simulink library "inp"  (R2021b)
settings: Solver=VariableStepAuto  StartTime=0.0  StopTime=10.0  RelTol=1e-3
undefined symbols (not defined in the file): C_TASK_5MS_S, FALSE, KINP_AcoreReadyToSlp_flg_ovrdflg, KINP_AcoreReadyToSlp_flg_ovrdval, KINP_AllowMovThd_OTA_enum_ovrdflg, KINP_AllowMovThd_OTA_enum_ovrdval, KINP_APSAngleTarget_Deg_ovrdflg, KINP_APSAngleTarget_Deg_ovrdval, KINP_APSDecReq_mps2_ovrdflg, KINP_APSDecReq_mps2_ovrdval, KINP_APSDecReqA_flg_ovrdflg, KINP_APSDecReqA_flg_ovrdval, KINP_APSDFLL_cm_ovrdflg, KINP_APSDFLL_cm_ovrdval, KINP_APSDFLR_cm_ovrdflg, KINP_APSDFLR_cm_ovrdval, KINP_APSDRLL_cm_ovrdflg, KINP_APSDRLL_cm_ovrdval, KINP_APSDRLR_cm_ovrdflg, KINP_APSDRLR_cm_ovrdval, KINP_APSExitCondition_enum_ovrdflg, KINP_APSExitCondition_enum_ovrdval, KINP_APSHWVer_enum_ovrdflg, KINP_APSHWVer_enum_ovrdval, KINP_APSProgressPCT_pct_ovrdflg, KINP_APSProgressPCT_pct_ovrdval, KINP_APSPwrReq_enum_ovrdflg, KINP_APSPwrReq_enum_ovrdval, KINP_APSReq_enum_ovrdflg, KINP_APSReq_enum_ovrdval, KINP_APSRQDisplay_enum_ovrdflg, KINP_APSRQDisplay_enum_ovrdval, KINP_APSRqEPASCtrl_flg_ovrdflg, KINP_APSRqEPASCtrl_flg_ovrdval, KINP_APSShiftPosnReq_enum_ovrdval, KINP_APSShiftPosnReq_enum_ovrflg, KINP_APSSpeedCMD_kph_ovrdval, KINP_APSSpeedCMD_kph_ovrflg, KINP_APSStaSystem_enum_ovrdflg, KINP_APSStaSystem_enum_ovrdval, KINP_APSSWVer_enum_ovrdflg, KINP_APSSWVer_enum_ovrdval, KINP_APSVMCReqA_flg_ovrdval, KINP_APSVMCReqA_flg_ovrflg, KINP_APSVRqEPASCtrl_flg_ovrdflg, KINP_APSVRqEPASCtrl_flg_ovrdval, KINP_AuxBattVolmV_mV_ovrdflg, KINP_AuxBattVolmV_mV_ovrdval, KINP_CAASSta_enum_ovrdflg, KINP_CAASSta_enum_ovrdval, KINP_CAASVMCReqA_flg_ovrdval, KINP_CAASVMCReqA_flg_ovrflg, KINP_CAN1BusOff_flg_ovrdflg, KINP_CAN1BusOff_flg_ovrdval, KINP_CAN2BusOff_flg_ovrdflg, KINP_CAN2BusOff_flg_ovrdval, KINP_CAN3BusOff_flg_ovrdflg, KINP_CAN3BusOff_flg_ovrdval, KINP_CAN4BusOff_flg_ovrdflg, KINP_CAN4BusOff_flg_ovrdval ... (+152)
libraries: FVT_lib x1035, hcu_lib x1
(part 25 of 33)

== system inp/INP/CAN4/SignalCheck/DKC1 ==
  BHAL_outputs : Inport
  inp_CanValid_bus : Inport  Port=2
  DKCKeyNumSta : FVT_lib/inp/can_signal_template  SystemSampleTime=-1  VariantActivationTime=update diagram  Latency=0  AutoFrameSizeCalculation=off
      link override defval: Value=KINP_DKCKeyNumSta_enum_defval
      link override ovrdflg: Value=KINP_DKCKeyNumSta_enum_ovrdflg
      link override ovrdval: Value=KINP_DKCKeyNumSta_enum_ovrdval
  DKCKeyTypeSta : FVT_lib/inp/can_signal_template  SystemSampleTime=-1  VariantActivationTime=update diagram  Latency=0  AutoFrameSizeCalculation=off
      link override defval: Value=KINP_DKCKeyTypeSta_enum_defval
      link override ovrdflg: Value=KINP_DKCKeyTypeSta_enum_ovrdflg
      link override ovrdval: Value=KINP_DKCKeyTypeSta_enum_ovrdval
  DKCPDkeyAreaRAPSSta : FVT_lib/inp/can_signal_template  SystemSampleTime=-1  VariantActivationTime=update diagram  Latency=0  AutoFrameSizeCalculation=off
      link override defval: Value=KINP_DKCPDkeyAreaRAPSSta_enum_defval
      link override ovrdflg: Value=KINP_DKCPDkeyAreaRAPSSta_enum_ovrdflg
      link override ovrdval: Value=KINP_DKCPDkeyAreaRAPSSta_enum_ovrdval
  DKCParkingModeCmd : FVT_lib/inp/can_signal_template  SystemSampleTime=-1  VariantActivationTime=update diagram  Latency=0  AutoFrameSizeCalculation=off
      link override defval: Value=KINP_DKCParkingModeCmd_enum_defval
      link override ovrdflg: Value=KINP_DKCParkingModeCmd_enum_ovrdflg
      link override ovrdval: Value=KINP_DKCParkingModeCmd_enum_ovrdval
  DKCReVehData : FVT_lib/inp/can_signal_template  SystemSampleTime=-1  VariantActivationTime=update diagram  Latency=0  AutoFrameSizeCalculation=off
      link override defval: Value=KINP_DKCReVehData_enum_defval
      link override ovrdflg: Value=KINP_DKCReVehData_enum_ovrdflg
      link override ovrdval: Value=KINP_DKCReVehData_enum_ovrdval
  PCommandToBCM : FVT_lib/inp/can_signal_template  SystemSampleTime=-1  VariantActivationTime=update diagram  Latency=0  AutoFrameSizeCalculation=off
      link override defval: Value=KINP_PCommandToBCM_enum_defval
      link override ovrdflg: Value=KINP_PCommandToBCM_enum_ovrdflg
      link override ovrdval: Value=KINP_PCommandToBCM_enum_ovrdval
  PCommandToPTG : FVT_lib/inp/can_signal_template  SystemSampleTime=-1  VariantActivationTime=update diagram  Latency=0  AutoFrameSizeCalculation=off
      link override defval: Value=KINP_PCommandToPTG_enum_defval
      link override ovrdflg: Value=KINP_PCommandToPTG_enum_ovrdflg
      link override ovrdval: Value=KINP_PCommandToPTG_enum_ovrdval
  PDKeyAreaLockUnlock : FVT_lib/inp/can_signal_template  SystemSampleTime=-1  VariantActivationTime=update diagram  Latency=0  AutoFrameSizeCalculation=off
      link override defval: Value=KINP_PDKeyAreaLockUnlock_enum_defval
      link override ovrdflg: Value=KINP_PDKeyAreaLockUnlock_enum_ovrdflg
      link override ovrdval: Value=KINP_PDKeyAreaLockUnlock_enum_ovrdval
  PDKeyAreaPS : FVT_lib/inp/can_signal_template  SystemSampleTime=-1  VariantActivationTime=update diagram  Latency=0  AutoFrameSizeCalculation=off
      link override defval: Value=KINP_PDKeyAreaPS_enum_defval
      link override ovrdflg: Value=KINP_PDKeyAreaPS_enum_ovrdflg
      link override ovrdval: Value=KINP_PDKeyAreaPS_enum_ovrdval
  PDKeyAreaPTG : FVT_lib/inp/can_signal_template  SystemSampleTime=-1  VariantActivationTime=update diagram  Latency=0  AutoFrameSizeCalculation=off
      link override defval: Value=KINP_PDKeyAreaPTG_enum_defval
      link override ovrdflg: Value=KINP_PDKeyAreaPTG_enum_ovrdflg
      link override ovrdval: Value=KINP_PDKeyAreaPTG_enum_ovrdval
  PDKeyWelcome : FVT_lib/inp/can_signal_template  SystemSampleTime=-1  VariantActivationTime=update diagram  Latency=0  AutoFrameSizeCalculation=off
      link override defval: Value=KINP_PDKeyWelcome_enum_defval
      link override ovrdflg: Value=KINP_PDKeyWelcome_enum_ovrdflg
      link override ovrdval: Value=KINP_PDKeyWelcome_enum_ovrdval
  PDkeyShowIVI : FVT_lib/inp/can_signal_template  SystemSampleTime=-1  VariantActivationTime=update diagram  Latency=0  AutoFrameSizeCalculation=off
      link override defval: Value=KINP_PDkeyShowIVI_enum_defval
      link override ovrdflg: Value=KINP_PDkeyShowIVI_enum_ovrdflg
      link override ovrdval: Value=KINP_PDkeyShowIVI_enum_ovrdval
  PKeyMiss : FVT_lib/inp/can_signal_template  SystemSampleTime=-1  VariantActivationTime=update diagram  Latency=0  AutoFrameSizeCalculation=off
      link override defval: Value=KINP_PKeyMiss_flg_defval
      link override ovrdflg: Value=KINP_PKeyMiss_flg_ovrdflg
      link override ovrdval: Value=KINP_PKeyMiss_flg_ovrdval
  PKeyMode : FVT_lib/inp/can_signal_template  SystemSampleTime=-1  VariantActivationTime=update diagram  Latency=0  AutoFrameSizeCalculation=off
      link override defval: Value=KINP_PKeyMode_enum_defval
      link override ovrdflg: Value=KINP_PKeyMode_enum_ovrdflg
      link override ovrdval: Value=KINP_PKeyMode_enum_ovrdval
  PUIDLowPower : FVT_lib/inp/can_signal_template  SystemSampleTime=-1  VariantActivationTime=update diagram  Latency=0  AutoFrameSizeCalculation=off
      link override defval: Value=KINP_PUIDLowPower_flg_defval
      link override ovrdflg: Value=KINP_PUIDLowPower_flg_ovrdflg
      link override ovrdval: Value=KINP_PUIDLowPower_flg_ovrdval
  Terminator_{1..15} (15 alike) : Terminator
  True_VHAL_DKCKeyNumSta_enum : Constant  Value=TRUE  OutDataTypeStr=boolean
  True_VHAL_DKCKeyTypeSta_enum : Constant  Value=TRUE  OutDataTypeStr=boolean
  True_VHAL_DKCPDkeyAreaRAPSSta_enum : Constant  Value=TRUE  OutDataTypeStr=boolean
  True_VHAL_DKCParkingModeCmd_enum : Constant  Value=TRUE  OutDataTypeStr=boolean
  True_VHAL_DKCReVehData_enum : Constant  Value=TRUE  OutDataTypeStr=boolean
  True_VHAL_PCommandToBCM_enum : Constant  Value=TRUE  OutDataTypeStr=boolean
  True_VHAL_PCommandToPTG_enum : Constant  Value=TRUE  OutDataTypeStr=boolean
  True_VHAL_PDKeyAreaLockUnlock_enum : Constant  Value=TRUE  OutDataTypeStr=boolean
  True_VHAL_PDKeyAreaPS_enum : Constant  Value=TRUE  OutDataTypeStr=boolean
  True_VHAL_PDKeyAreaPTG_enum : Constant  Value=TRUE  OutDataTypeStr=boolean
  True_VHAL_PDKeyWelcome_enum : Constant  Value=TRUE  OutDataTypeStr=boolean
  True_VHAL_PDkeyShowIVI_enum : Constant  Value=TRUE  OutDataTypeStr=boolean
  True_VHAL_PKeyMiss_flg : Constant  Value=TRUE  OutDataTypeStr=boolean
  True_VHAL_PKeyMode_enum : Constant  Value=TRUE  OutDataTypeStr=boolean
  True_VHAL_PUIDLowPower_flg : Constant  Value=TRUE  OutDataTypeStr=boolean
  slr1_{1..15} (15 alike) : BusSelector  OutputSignals=VINP_CANMsgValidDKC1_flg
  slr_VHAL_DKCKeyNumSta_enum : BusSelector  OutputSignals=VHAL_DKCKeyNumSta_enum
  slr_VHAL_DKCKeyTypeSta_enum : BusSelector  OutputSignals=VHAL_DKCKeyTypeSta_enum
  slr_VHAL_DKCPDkeyAreaRAPSSta_enum : BusSelector  OutputSignals=VHAL_DKCPDkeyAreaRAPSSta_enum
  slr_VHAL_DKCParkingModeCmd_enum : BusSelector  OutputSignals=VHAL_DKCParkingModeCmd_enum
  slr_VHAL_DKCReVehData_enum : BusSelector  OutputSignals=VHAL_DKCReVehData_enum
  slr_VHAL_PCommandToBCM_enum : BusSelector  OutputSignals=VHAL_PCommandToBCM_enum
  slr_VHAL_PCommandToPTG_enum : BusSelector  OutputSignals=VHAL_PCommandToPTG_enum
  slr_VHAL_PDKeyAreaLockUnlock_enum : BusSelector  OutputSignals=VHAL_PDKeyAreaLockUnlock_enum
  slr_VHAL_PDKeyAreaPS_enum : BusSelector  OutputSignals=VHAL_PDKeyAreaPS_enum
  slr_VHAL_PDKeyAreaPTG_enum : BusSelector  OutputSignals=VHAL_PDKeyAreaPTG_enum
  slr_VHAL_PDKeyWelcome_enum : BusSelector  OutputSignals=VHAL_PDKeyWelcome_enum
  slr_VHAL_PDkeyShowIVI_enum : BusSelector  OutputSignals=VHAL_PDkeyShowIVI_enum
  slr_VHAL_PKeyMiss_flg : BusSelector  OutputSignals=VHAL_PKeyMiss_flg
  slr_VHAL_PKeyMode_enum : BusSelector  OutputSignals=VHAL_PKeyMode_enum
  slr_VHAL_PUIDLowPower_flg : BusSelector  OutputSignals=VHAL_PUIDLowPower_flg
  VINP_DKCKeyNumSta_enum : Outport
  VINP_DKCKeyTypeSta_enum : Outport  Port=2
  VINP_DKCPDkeyAreaRAPSSta_enum : Outport  Port=3
  VINP_DKCParkingModeCmd_enum : Outport  Port=4
  VINP_DKCReVehData_enum : Outport  Port=5
  VINP_PCommandToBCM_enum : Outport  Port=6
  VINP_PCommandToPTG_enum : Outport  Port=7
  VINP_PDKeyAreaLockUnlock_enum : Outport  Port=8
  VINP_PDKeyAreaPS_enum : Outport  Port=9
  VINP_PDKeyAreaPTG_enum : Outport  Port=10
  VINP_PDKeyWelcome_enum : Outport  Port=11
  VINP_PDkeyShowIVI_enum : Outport  Port=12
  VINP_PKeyMiss_flg : Outport  Port=13
  VINP_PKeyMode_enum : Outport  Port=14
  VINP_PUIDLowPower_flg : Outport  Port=15
  wires:
  BHAL_outputs/1 -> [BHAL_outputs]
  inp_CanValid_bus/1 -> [inp_CanValid_bus]
  [BHAL_outputs] -> slr_VHAL_DKCKeyNumSta_enum/1
  slr_VHAL_DKCKeyNumSta_enum/1 -> DKCKeyNumSta/1  "<VHAL_DKCKeyNumSta_enum>"
  True_VHAL_DKCKeyNumSta_enum/1 -> DKCKeyNumSta/2
  [inp_CanValid_bus] -> slr1_1/1
  slr1_1/1 -> DKCKeyNumSta/3  "<VINP_CANMsgValidDKC1_flg>"
  DKCKeyNumSta/1 -> VINP_DKCKeyNumSta_enum/1  "VINP_DKCKeyNumSta_enum"
  DKCKeyNumSta/2 -> Terminator_1/1
  [BHAL_outputs] -> slr_VHAL_DKCKeyTypeSta_enum/1
  slr_VHAL_DKCKeyTypeSta_enum/1 -> DKCKeyTypeSta/1  "<VHAL_DKCKeyTypeSta_enum>"
  True_VHAL_DKCKeyTypeSta_enum/1 -> DKCKeyTypeSta/2
  [inp_CanValid_bus] -> slr1_2/1
  slr1_2/1 -> DKCKeyTypeSta/3  "<VINP_CANMsgValidDKC1_flg>"
  DKCKeyTypeSta/1 -> VINP_DKCKeyTypeSta_enum/1  "VINP_DKCKeyTypeSta_enum"
  DKCKeyTypeSta/2 -> Terminator_2/1
  [BHAL_outputs] -> slr_VHAL_DKCPDkeyAreaRAPSSta_enum/1
  slr_VHAL_DKCPDkeyAreaRAPSSta_enum/1 -> DKCPDkeyAreaRAPSSta/1  "<VHAL_DKCPDkeyAreaRAPSSta_enum>"
  True_VHAL_DKCPDkeyAreaRAPSSta_enum/1 -> DKCPDkeyAreaRAPSSta/2
  [inp_CanValid_bus] -> slr1_3/1
  slr1_3/1 -> DKCPDkeyAreaRAPSSta/3  "<VINP_CANMsgValidDKC1_flg>"
  DKCPDkeyAreaRAPSSta/1 -> VINP_DKCPDkeyAreaRAPSSta_enum/1  "VINP_DKCPDkeyAreaRAPSSta_enum"
  DKCPDkeyAreaRAPSSta/2 -> Terminator_3/1
  [BHAL_outputs] -> slr_VHAL_DKCParkingModeCmd_enum/1
  slr_VHAL_DKCParkingModeCmd_enum/1 -> DKCParkingModeCmd/1  "<VHAL_DKCParkingModeCmd_enum>"
  True_VHAL_DKCParkingModeCmd_enum/1 -> DKCParkingModeCmd/2
  [inp_CanValid_bus] -> slr1_4/1
  slr1_4/1 -> DKCParkingModeCmd/3  "<VINP_CANMsgValidDKC1_flg>"
  DKCParkingModeCmd/1 -> VINP_DKCParkingModeCmd_enum/1  "VINP_DKCParkingModeCmd_enum"
  DKCParkingModeCmd/2 -> Terminator_4/1
  [BHAL_outputs] -> slr_VHAL_DKCReVehData_enum/1
  slr_VHAL_DKCReVehData_enum/1 -> DKCReVehData/1  "<VHAL_DKCReVehData_enum>"
  True_VHAL_DKCReVehData_enum/1 -> DKCReVehData/2
  [inp_CanValid_bus] -> slr1_5/1
  slr1_5/1 -> DKCReVehData/3  "<VINP_CANMsgValidDKC1_flg>"
  DKCReVehData/1 -> VINP_DKCReVehData_enum/1  "VINP_DKCReVehData_enum"
  DKCReVehData/2 -> Terminator_5/1
  [BHAL_outputs] -> slr_VHAL_PCommandToBCM_enum/1
  slr_VHAL_PCommandToBCM_enum/1 -> PCommandToBCM/1  "<VHAL_PCommandToBCM_enum>"
  True_VHAL_PCommandToBCM_enum/1 -> PCommandToBCM/2
  [inp_CanValid_bus] -> slr1_6/1
  slr1_6/1 -> PCommandToBCM/3  "<VINP_CANMsgValidDKC1_flg>"
  PCommandToBCM/1 -> VINP_PCommandToBCM_enum/1  "VINP_PCommandToBCM_enum"
  PCommandToBCM/2 -> Terminator_6/1
  [BHAL_outputs] -> slr_VHAL_PCommandToPTG_enum/1
  slr_VHAL_PCommandToPTG_enum/1 -> PCommandToPTG/1  "<VHAL_PCommandToPTG_enum>"
  True_VHAL_PCommandToPTG_enum/1 -> PCommandToPTG/2
  [inp_CanValid_bus] -> slr1_7/1
  slr1_7/1 -> PCommandToPTG/3  "<VINP_CANMsgValidDKC1_flg>"
  PCommandToPTG/1 -> VINP_PCommandToPTG_enum/1  "VINP_PCommandToPTG_enum"
  PCommandToPTG/2 -> Terminator_7/1
  [BHAL_outputs] -> slr_VHAL_PDKeyAreaLockUnlock_enum/1
  slr_VHAL_PDKeyAreaLockUnlock_enum/1 -> PDKeyAreaLockUnlock/1  "<VHAL_PDKeyAreaLockUnlock_enum>"
  True_VHAL_PDKeyAreaLockUnlock_enum/1 -> PDKeyAreaLockUnlock/2
  [inp_CanValid_bus] -> slr1_8/1
  slr1_8/1 -> PDKeyAreaLockUnlock/3  "<VINP_CANMsgValidDKC1_flg>"
  PDKeyAreaLockUnlock/1 -> VINP_PDKeyAreaLockUnlock_enum/1  "VINP_PDKeyAreaLockUnlock_enum"
  PDKeyAreaLockUnlock/2 -> Terminator_8/1
  [BHAL_outputs] -> slr_VHAL_PDKeyAreaPS_enum/1
  slr_VHAL_PDKeyAreaPS_enum/1 -> PDKeyAreaPS/1  "<VHAL_PDKeyAreaPS_enum>"
  True_VHAL_PDKeyAreaPS_enum/1 -> PDKeyAreaPS/2
  [inp_CanValid_bus] -> slr1_9/1
  slr1_9/1 -> PDKeyAreaPS/3  "<VINP_CANMsgValidDKC1_flg>"
  PDKeyAreaPS/1 -> VINP_PDKeyAreaPS_enum/1  "VINP_PDKeyAreaPS_enum"
  PDKeyAreaPS/2 -> Terminator_9/1
  [BHAL_outputs] -> slr_VHAL_PDKeyAreaPTG_enum/1
  slr_VHAL_PDKeyAreaPTG_enum/1 -> PDKeyAreaPTG/1  "<VHAL_PDKeyAreaPTG_enum>"
  True_VHAL_PDKeyAreaPTG_enum/1 -> PDKeyAreaPTG/2
  [inp_CanValid_bus] -> slr1_10/1
  slr1_10/1 -> PDKeyAreaPTG/3  "<VINP_CANMsgValidDKC1_flg>"
  PDKeyAreaPTG/1 -> VINP_PDKeyAreaPTG_enum/1  "VINP_PDKeyAreaPTG_enum"
  PDKeyAreaPTG/2 -> Terminator_10/1
  [BHAL_outputs] -> slr_VHAL_PDKeyWelcome_enum/1
  slr_VHAL_PDKeyWelcome_enum/1 -> PDKeyWelcome/1  "<VHAL_PDKeyWelcome_enum>"
  True_VHAL_PDKeyWelcome_enum/1 -> PDKeyWelcome/2
  [inp_CanValid_bus] -> slr1_11/1
  slr1_11/1 -> PDKeyWelcome/3  "<VINP_CANMsgValidDKC1_flg>"
  PDKeyWelcome/1 -> VINP_PDKeyWelcome_enum/1  "VINP_PDKeyWelcome_enum"
  PDKeyWelcome/2 -> Terminator_11/1
  [BHAL_outputs] -> slr_VHAL_PDkeyShowIVI_enum/1
  slr_VHAL_PDkeyShowIVI_enum/1 -> PDkeyShowIVI/1  "<VHAL_PDkeyShowIVI_enum>"
  True_VHAL_PDkeyShowIVI_enum/1 -> PDkeyShowIVI/2
  [inp_CanValid_bus] -> slr1_12/1
  slr1_12/1 -> PDkeyShowIVI/3  "<VINP_CANMsgValidDKC1_flg>"
  PDkeyShowIVI/1 -> VINP_PDkeyShowIVI_enum/1  "VINP_PDkeyShowIVI_enum"
  PDkeyShowIVI/2 -> Terminator_12/1
  [BHAL_outputs] -> slr_VHAL_PKeyMiss_flg/1
  slr_VHAL_PKeyMiss_flg/1 -> PKeyMiss/1  "<VHAL_PKeyMiss_flg>"
  True_VHAL_PKeyMiss_flg/1 -> PKeyMiss/2
  [inp_CanValid_bus] -> slr1_13/1
  slr1_13/1 -> PKeyMiss/3  "<VINP_CANMsgValidDKC1_flg>"
  PKeyMiss/1 -> VINP_PKeyMiss_flg/1  "VINP_PKeyMiss_flg"
  PKeyMiss/2 -> Terminator_13/1
  [BHAL_outputs] -> slr_VHAL_PKeyMode_enum/1
  slr_VHAL_PKeyMode_enum/1 -> PKeyMode/1  "<VHAL_PKeyMode_enum>"
  True_VHAL_PKeyMode_enum/1 -> PKeyMode/2
  [inp_CanValid_bus] -> slr1_14/1
  slr1_14/1 -> PKeyMode/3  "<VINP_CANMsgValidDKC1_flg>"
  PKeyMode/1 -> VINP_PKeyMode_enum/1  "VINP_PKeyMode_enum"
  PKeyMode/2 -> Terminator_14/1
  [BHAL_outputs] -> slr_VHAL_PUIDLowPower_flg/1
  slr_VHAL_PUIDLowPower_flg/1 -> PUIDLowPower/1  "<VHAL_PUIDLowPower_flg>"
  True_VHAL_PUIDLowPower_flg/1 -> PUIDLowPower/2
  [inp_CanValid_bus] -> slr1_15/1
  slr1_15/1 -> PUIDLowPower/3  "<VINP_CANMsgValidDKC1_flg>"
  PUIDLowPower/1 -> VINP_PUIDLowPower_flg/1  "VINP_PUIDLowPower_flg"
  PUIDLowPower/2 -> Terminator_15/1

== system inp/INP/CAN4/SignalCheck/DKC2 ==
  BHAL_outputs : Inport
  inp_CanValid_bus : Inport  Port=2
  EncryptionDATA063 : FVT_lib/inp/can_signal_template  SystemSampleTime=-1  VariantActivationTime=update diagram  Latency=0  AutoFrameSizeCalculation=off
      link override defval: Value=KINP_EncryptionDATA063_enum_defval
      link override ovrdflg: Value=KINP_EncryptionDATA063_enum_ovrdflg
      link override ovrdval: Value=KINP_EncryptionDATA063_enum_ovrdval
  EncryptionDATA64127 : FVT_lib/inp/can_signal_template  SystemSampleTime=-1  VariantActivationTime=update diagram  Latency=0  AutoFrameSizeCalculation=off
      link override defval: Value=KINP_EncryptionDATA64127_enum_defval
      link override ovrdflg: Value=KINP_EncryptionDATA64127_enum_ovrdflg
      link override ovrdval: Value=KINP_EncryptionDATA64127_enum_ovrdval
  RandomNumberX : FVT_lib/inp/can_signal_template  SystemSampleTime=-1  VariantActivationTime=update diagram  Latency=0  AutoFrameSizeCalculation=off
      link override defval: Value=KINP_RandomNumberX_enum_defval
      link override ovrdflg: Value=KINP_RandomNumberX_enum_ovrdflg
      link override ovrdval: Value=KINP_RandomNumberX_enum_ovrdval
  Terminator_1 : Terminator
  Terminator_2 : Terminator
  Terminator_3 : Terminator
  True_VHAL_EncryptionDATA063_enum : Constant  Value=TRUE  OutDataTypeStr=boolean
  True_VHAL_EncryptionDATA64127_enum : Constant  Value=TRUE  OutDataTypeStr=boolean
  True_VHAL_RandomNumberX_enum : Constant  Value=TRUE  OutDataTypeStr=boolean
  slr1_1 : BusSelector  OutputSignals=VINP_CANMsgValidDKC2_flg
  slr1_2 : BusSelector  OutputSignals=VINP_CANMsgValidDKC2_flg
  slr1_3 : BusSelector  OutputSignals=VINP_CANMsgValidDKC2_flg
  slr_VHAL_EncryptionDATA063_enum : BusSelector  OutputSignals=VHAL_EncryptionDATA063_enum
  slr_VHAL_EncryptionDATA64127_enum : BusSelector  OutputSignals=VHAL_EncryptionDATA64127_enum
  slr_VHAL_RandomNumberX_enum : BusSelector  OutputSignals=VHAL_RandomNumberX_enum
  VINP_EncryptionDATA063_enum : Outport
  VINP_EncryptionDATA64127_enum : Outport  Port=2
  VINP_RandomNumberX_enum : Outport  Port=3
  wires:
  BHAL_outputs/1 -> [BHAL_outputs]
  inp_CanValid_bus/1 -> [inp_CanValid_bus]
  [BHAL_outputs] -> slr_VHAL_EncryptionDATA063_enum/1
  slr_VHAL_EncryptionDATA063_enum/1 -> EncryptionDATA063/1  "<VHAL_EncryptionDATA063_enum>"
  True_VHAL_EncryptionDATA063_enum/1 -> EncryptionDATA063/2
  [inp_CanValid_bus] -> slr1_1/1
  slr1_1/1 -> EncryptionDATA063/3  "<VINP_CANMsgValidDKC2_flg>"
  EncryptionDATA063/1 -> VINP_EncryptionDATA063_enum/1  "VINP_EncryptionDATA063_enum"
  EncryptionDATA063/2 -> Terminator_1/1
  [BHAL_outputs] -> slr_VHAL_EncryptionDATA64127_enum/1
  slr_VHAL_EncryptionDATA64127_enum/1 -> EncryptionDATA64127/1  "<VHAL_EncryptionDATA64127_enum>"
  True_VHAL_EncryptionDATA64127_enum/1 -> EncryptionDATA64127/2
  [inp_CanValid_bus] -> slr1_2/1
  slr1_2/1 -> EncryptionDATA64127/3  "<VINP_CANMsgValidDKC2_flg>"
  EncryptionDATA64127/1 -> VINP_EncryptionDATA64127_enum/1  "VINP_EncryptionDATA64127_enum"
  EncryptionDATA64127/2 -> Terminator_2/1
  [BHAL_outputs] -> slr_VHAL_RandomNumberX_enum/1
  slr_VHAL_RandomNumberX_enum/1 -> RandomNumberX/1  "<VHAL_RandomNumberX_enum>"
  True_VHAL_RandomNumberX_enum/1 -> RandomNumberX/2
  [inp_CanValid_bus] -> slr1_3/1
  slr1_3/1 -> RandomNumberX/3  "<VINP_CANMsgValidDKC2_flg>"
  RandomNumberX/1 -> VINP_RandomNumberX_enum/1  "VINP_RandomNumberX_enum"
  RandomNumberX/2 -> Terminator_3/1

== system inp/INP/CAN4/SignalCheck/PTG1 ==
  BHAL_outputs : Inport
  inp_CanValid_bus : Inport  Port=2
  PTGActiveSta : FVT_lib/inp/can_signal_template  SystemSampleTime=-1  VariantActivationTime=update diagram  Latency=0  AutoFrameSizeCalculation=off
      link override defval: Value=KINP_PTGActiveSta_enum_defval
      link override ovrdflg: Value=KINP_PTGActiveSta_enum_ovrdflg
      link override ovrdval: Value=KINP_PTGActiveSta_enum_ovrdval
  PTGAutoStaus : FVT_lib/inp/can_signal_template  SystemSampleTime=-1  VariantActivationTime=update diagram  Latency=0  AutoFrameSizeCalculation=off
      link override defval: Value=KINP_PTGAutoStaus_flg_defval
      link override ovrdflg: Value=KINP_PTGAutoStaus_flg_ovrdflg
      link override ovrdval: Value=KINP_PTGAutoStaus_flg_ovrdval
  PTGExist : FVT_lib/inp/can_signal_template  SystemSampleTime=-1  VariantActivationTime=update diagram  Latency=0  AutoFrameSizeCalculation=off
      link override defval: Value=KINP_PTGExist_flg_defval
      link override ovrdflg: Value=KINP_PTGExist_flg_ovrdflg
      link override ovrdval: Value=KINP_PTGExist_flg_ovrdval
  PTGHWVer : FVT_lib/inp/can_signal_template  SystemSampleTime=-1  VariantActivationTime=update diagram  Latency=0  AutoFrameSizeCalculation=off
      link override defval: Value=KINP_PTGHWVer_enum_defval
      link override ovrdflg: Value=KINP_PTGHWVer_enum_ovrdflg
      link override ovrdval: Value=KINP_PTGHWVer_enum_ovrdval
  PTGInnerSW2 : FVT_lib/inp/can_signal_template  SystemSampleTime=-1  VariantActivationTime=update diagram  Latency=0  AutoFrameSizeCalculation=off
      link override defval: Value=KINP_PTGInnerSW2_enum_defval
      link override ovrdflg: Value=KINP_PTGInnerSW2_enum_ovrdflg
      link override ovrdval: Value=KINP_PTGInnerSW2_enum_ovrdval
  PTGIsSetHeight : FVT_lib/inp/can_signal_template  SystemSampleTime=-1  VariantActivationTime=update diagram  Latency=0  AutoFrameSizeCalculation=off
      link override defval: Value=KINP_PTGIsSetHeight_flg_defval
      link override ovrdflg: Value=KINP_PTGIsSetHeight_flg_ovrdflg
      link override ovrdval: Value=KINP_PTGIsSetHeight_flg_ovrdval
  PTGOpenRatio : FVT_lib/inp/can_signal_template  SystemSampleTime=-1  VariantActivationTime=update diagram  Latency=0  AutoFrameSizeCalculation=off
      link override defval: Value=KINP_PTGOpenRatio_pct_defval
      link override ovrdflg: Value=KINP_PTGOpenRatio_pct_ovrdflg
      link override ovrdval: Value=KINP_PTGOpenRatio_pct_ovrdval
  PTGRDILSta : FVT_lib/inp/can_signal_template  SystemSampleTime=-1  VariantActivationTime=update diagram  Latency=0  AutoFrameSizeCalculation=off
      link override defval: Value=KINP_PTGRDILSta_enum_defval
      link override ovrdflg: Value=KINP_PTGRDILSta_enum_ovrdflg
      link override ovrdval: Value=KINP_PTGRDILSta_enum_ovrdval
  PTGSWVer : FVT_lib/inp/can_signal_template  SystemSampleTime=-1  VariantActivationTime=update diagram  Latency=0  AutoFrameSizeCalculation=off
      link override defval: Value=KINP_PTGSWVer_enum_defval
      link override ovrdflg: Value=KINP_PTGSWVer_enum_ovrdflg
      link override ovrdval: Value=KINP_PTGSWVer_enum_ovrdval
  PTGSysSta : FVT_lib/inp/can_signal_template  SystemSampleTime=-1  VariantActivationTime=update diagram  Latency=0  AutoFrameSizeCalculation=off
      link override defval: Value=KINP_PTGSysSta_enum_defval
      link override ovrdflg: Value=KINP_PTGSysSta_enum_ovrdflg
      link override ovrdval: Value=KINP_PTGSysSta_enum_ovrdval
  Terminator_{1..10} (10 alike) : Terminator
  True_VHAL_PTGActiveSta_enum : Constant  Value=TRUE  OutDataTypeStr=boolean
  True_VHAL_PTGAutoStaus_flg : Constant  Value=TRUE  OutDataTypeStr=boolean
  True_VHAL_PTGExist_flg : Constant  Value=TRUE  OutDataTypeStr=boolean
  True_VHAL_PTGHWVer_enum : Constant  Value=TRUE  OutDataTypeStr=boolean
  True_VHAL_PTGInnerSW2_enum : Constant  Value=TRUE  OutDataTypeStr=boolean
  True_VHAL_PTGIsSetHeight_flg : Constant  Value=TRUE  OutDataTypeStr=boolean
  True_VHAL_PTGOpenRatio_pct : Constant  Value=TRUE  OutDataTypeStr=boolean
  True_VHAL_PTGRDILSta_enum : Constant  Value=TRUE  OutDataTypeStr=boolean
  True_VHAL_PTGSWVer_enum : Constant  Value=TRUE  OutDataTypeStr=boolean
  True_VHAL_PTGSysSta_enum : Constant  Value=TRUE  OutDataTypeStr=boolean
  slr1_{1..10} (10 alike) : BusSelector  OutputSignals=VINP_CANMsgValidPTG1_flg
  slr_VHAL_PTGActiveSta_enum : BusSelector  OutputSignals=VHAL_PTGActiveSta_enum
  slr_VHAL_PTGAutoStaus_flg : BusSelector  OutputSignals=VHAL_PTGAutoStaus_flg
  slr_VHAL_PTGExist_flg : BusSelector  OutputSignals=VHAL_PTGExist_flg
  slr_VHAL_PTGHWVer_enum : BusSelector  OutputSignals=VHAL_PTGHWVer_enum
  slr_VHAL_PTGInnerSW2_enum : BusSelector  OutputSignals=VHAL_PTGInnerSW2_enum
  slr_VHAL_PTGIsSetHeight_flg : BusSelector  OutputSignals=VHAL_PTGIsSetHeight_flg
  slr_VHAL_PTGOpenRatio_pct : BusSelector  OutputSignals=VHAL_PTGOpenRatio_pct
  slr_VHAL_PTGRDILSta_enum : BusSelector  OutputSignals=VHAL_PTGRDILSta_enum
  slr_VHAL_PTGSWVer_enum : BusSelector  OutputSignals=VHAL_PTGSWVer_enum
  slr_VHAL_PTGSysSta_enum : BusSelector  OutputSignals=VHAL_PTGSysSta_enum
  VINP_PTGActiveSta_enum : Outport
  VINP_PTGAutoStaus_flg : Outport  Port=2
  VINP_PTGExist_flg : Outport  Port=3
  VINP_PTGHWVer_enum : Outport  Port=4
  VINP_PTGInnerSW2_enum : Outport  Port=5
  VINP_PTGIsSetHeight_flg : Outport  Port=6
  VINP_PTGOpenRatio_pct : Outport  Port=7
  VINP_PTGRDILSta_enum : Outport  Port=8
  VINP_PTGSWVer_enum : Outport  Port=9
  VINP_PTGSysSta_enum : Outport  Port=10
  wires:
  BHAL_outputs/1 -> [BHAL_outputs]
  inp_CanValid_bus/1 -> [inp_CanValid_bus]
  [BHAL_outputs] -> slr_VHAL_PTGActiveSta_enum/1
  slr_VHAL_PTGActiveSta_enum/1 -> PTGActiveSta/1  "<VHAL_PTGActiveSta_enum>"
  True_VHAL_PTGActiveSta_enum/1 -> PTGActiveSta/2
  [inp_CanValid_bus] -> slr1_1/1
  slr1_1/1 -> PTGActiveSta/3  "<VINP_CANMsgValidPTG1_flg>"
  PTGActiveSta/1 -> VINP_PTGActiveSta_enum/1  "VINP_PTGActiveSta_enum"
  PTGActiveSta/2 -> Terminator_1/1
  [BHAL_outputs] -> slr_VHAL_PTGAutoStaus_flg/1
  slr_VHAL_PTGAutoStaus_flg/1 -> PTGAutoStaus/1  "<VHAL_PTGAutoStaus_flg>"
  True_VHAL_PTGAutoStaus_flg/1 -> PTGAutoStaus/2
  [inp_CanValid_bus] -> slr1_2/1
  slr1_2/1 -> PTGAutoStaus/3  "<VINP_CANMsgValidPTG1_flg>"
  PTGAutoStaus/1 -> VINP_PTGAutoStaus_flg/1  "VINP_PTGAutoStaus_flg"
  PTGAutoStaus/2 -> Terminator_2/1
  [BHAL_outputs] -> slr_VHAL_PTGExist_flg/1
  slr_VHAL_PTGExist_flg/1 -> PTGExist/1  "<VHAL_PTGExist_flg>"
  True_VHAL_PTGExist_flg/1 -> PTGExist/2
  [inp_CanValid_bus] -> slr1_3/1
  slr1_3/1 -> PTGExist/3  "<VINP_CANMsgValidPTG1_flg>"
  PTGExist/1 -> VINP_PTGExist_flg/1  "VINP_PTGExist_flg"
  PTGExist/2 -> Terminator_3/1
  [BHAL_outputs] -> slr_VHAL_PTGHWVer_enum/1
  slr_VHAL_PTGHWVer_enum/1 -> PTGHWVer/1  "<VHAL_PTGHWVer_enum>"
  True_VHAL_PTGHWVer_enum/1 -> PTGHWVer/2
  [inp_CanValid_bus] -> slr1_4/1
  slr1_4/1 -> PTGHWVer/3  "<VINP_CANMsgValidPTG1_flg>"
  PTGHWVer/1 -> VINP_PTGHWVer_enum/1  "VINP_PTGHWVer_enum"
  PTGHWVer/2 -> Terminator_4/1
  [BHAL_outputs] -> slr_VHAL_PTGInnerSW2_enum/1
  slr_VHAL_PTGInnerSW2_enum/1 -> PTGInnerSW2/1  "<VHAL_PTGInnerSW2_enum>"
  True_VHAL_PTGInnerSW2_enum/1 -> PTGInnerSW2/2
  [inp_CanValid_bus] -> slr1_5/1
  slr1_5/1 -> PTGInnerSW2/3  "<VINP_CANMsgValidPTG1_flg>"
  PTGInnerSW2/1 -> VINP_PTGInnerSW2_enum/1  "VINP_PTGInnerSW2_enum"
  PTGInnerSW2/2 -> Terminator_5/1
  [BHAL_outputs] -> slr_VHAL_PTGIsSetHeight_flg/1
  slr_VHAL_PTGIsSetHeight_flg/1 -> PTGIsSetHeight/1  "<VHAL_PTGIsSetHeight_flg>"
  True_VHAL_PTGIsSetHeight_flg/1 -> PTGIsSetHeight/2
  [inp_CanValid_bus] -> slr1_6/1
  slr1_6/1 -> PTGIsSetHeight/3  "<VINP_CANMsgValidPTG1_flg>"
  PTGIsSetHeight/1 -> VINP_PTGIsSetHeight_flg/1  "VINP_PTGIsSetHeight_flg"
  PTGIsSetHeight/2 -> Terminator_6/1
  [BHAL_outputs] -> slr_VHAL_PTGOpenRatio_pct/1
  slr_VHAL_PTGOpenRatio_pct/1 -> PTGOpenRatio/1  "<VHAL_PTGOpenRatio_pct>"
  True_VHAL_PTGOpenRatio_pct/1 -> PTGOpenRatio/2
  [inp_CanValid_bus] -> slr1_7/1
  slr1_7/1 -> PTGOpenRatio/3  "<VINP_CANMsgValidPTG1_flg>"
  PTGOpenRatio/1 -> VINP_PTGOpenRatio_pct/1  "VINP_PTGOpenRatio_pct"
  PTGOpenRatio/2 -> Terminator_7/1
  [BHAL_outputs] -> slr_VHAL_PTGRDILSta_enum/1
  slr_VHAL_PTGRDILSta_enum/1 -> PTGRDILSta/1  "<VHAL_PTGRDILSta_enum>"
  True_VHAL_PTGRDILSta_enum/1 -> PTGRDILSta/2
  [inp_CanValid_bus] -> slr1_8/1
  slr1_8/1 -> PTGRDILSta/3  "<VINP_CANMsgValidPTG1_flg>"
  PTGRDILSta/1 -> VINP_PTGRDILSta_enum/1  "VINP_PTGRDILSta_enum"
  PTGRDILSta/2 -> Terminator_8/1
  [BHAL_outputs] -> slr_VHAL_PTGSWVer_enum/1
  slr_VHAL_PTGSWVer_enum/1 -> PTGSWVer/1  "<VHAL_PTGSWVer_enum>"
  True_VHAL_PTGSWVer_enum/1 -> PTGSWVer/2
  [inp_CanValid_bus] -> slr1_9/1
  slr1_9/1 -> PTGSWVer/3  "<VINP_CANMsgValidPTG1_flg>"
  PTGSWVer/1 -> VINP_PTGSWVer_enum/1  "VINP_PTGSWVer_enum"
  PTGSWVer/2 -> Terminator_9/1
  [BHAL_outputs] -> slr_VHAL_PTGSysSta_enum/1
  slr_VHAL_PTGSysSta_enum/1 -> PTGSysSta/1  "<VHAL_PTGSysSta_enum>"
  True_VHAL_PTGSysSta_enum/1 -> PTGSysSta/2
  [inp_CanValid_bus] -> slr1_10/1
  slr1_10/1 -> PTGSysSta/3  "<VINP_CANMsgValidPTG1_flg>"
  PTGSysSta/1 -> VINP_PTGSysSta_enum/1  "VINP_PTGSysSta_enum"
  PTGSysSta/2 -> Terminator_10/1

== system inp/INP/CAN4/SignalCheck/ZONE_DR1 ==
  BHAL_outputs : Inport
  inp_CanValid_bus : Inport  Port=2
  DrLockSta : FVT_lib/inp/can_signal_template  SystemSampleTime=-1  VariantActivationTime=update diagram  Latency=0  AutoFrameSizeCalculation=off
      link override defval: Value=KINP_DrLockSta_flg_defval
      link override ovrdflg: Value=KINP_DrLockSta_flg_ovrdflg
      link override ovrdval: Value=KINP_DrLockSta_flg_ovrdval
  MIRRORFOLDSW : FVT_lib/inp/can_signal_template  SystemSampleTime=-1  VariantActivationTime=update diagram  Latency=0  AutoFrameSizeCalculation=off
      link override defval: Value=KINP_MIRRORFOLDSW_flg_defval
      link override ovrdflg: Value=KINP_MIRRORFOLDSW_flg_ovrdflg
      link override ovrdval: Value=KINP_MIRRORFOLDSW_flg_ovrdval
  RLTurnLPErr : FVT_lib/inp/can_signal_template  SystemSampleTime=-1  VariantActivationTime=update diagram  Latency=0  AutoFrameSizeCalculation=off
      link override defval: Value=KINP_RLTurnLPErr_flg_defval
      link override ovrdflg: Value=KINP_RLTurnLPErr_flg_ovrdflg
      link override ovrdval: Value=KINP_RLTurnLPErr_flg_ovrdval
  RLTurnLampC : FVT_lib/inp/can_signal_template  SystemSampleTime=-1  VariantActivationTime=update diagram  Latency=0  AutoFrameSizeCalculation=off
      link override defval: Value=KINP_RLTurnLampC_mA_defval
      link override ovrdflg: Value=KINP_RLTurnLampC_mA_ovrdflg
      link override ovrdval: Value=KINP_RLTurnLampC_mA_ovrdval
  RRTurnLPErr : FVT_lib/inp/can_signal_template  SystemSampleTime=-1  VariantActivationTime=update diagram  Latency=0  AutoFrameSizeCalculation=off
      link override defval: Value=KINP_RRTurnLPErr_flg_defval
      link override ovrdflg: Value=KINP_RRTurnLPErr_flg_ovrdflg
      link override ovrdval: Value=KINP_RRTurnLPErr_flg_ovrdval
  RRTurnLampC : FVT_lib/inp/can_signal_template  SystemSampleTime=-1  VariantActivationTime=update diagram  Latency=0  AutoFrameSizeCalculation=off
      link override defval: Value=KINP_RRTurnLampC_mA_defval
      link override ovrdflg: Value=KINP_RRTurnLampC_mA_ovrdflg
      link override ovrdval: Value=KINP_RRTurnLampC_mA_ovrdval
  RWiperAS : FVT_lib/inp/can_signal_template  SystemSampleTime=-1  VariantActivationTime=update diagram  Latency=0  AutoFrameSizeCalculation=off
      link override defval: Value=KINP_RWiperAS_flg_defval
      link override ovrdflg: Value=KINP_RWiperAS_flg_ovrdflg
      link override ovrdval: Value=KINP_RWiperAS_flg_ovrdval
  RWiperProtection : FVT_lib/inp/can_signal_template  SystemSampleTime=-1  VariantActivationTime=update diagram  Latency=0  AutoFrameSizeCalculation=off
      link override defval: Value=KINP_RWiperProtection_flg_defval
      link override ovrdflg: Value=KINP_RWiperProtection_flg_ovrdflg
      link override ovrdval: Value=KINP_RWiperProtection_flg_ovrdval
  Terminator_{1..8} (8 alike) : Terminator
  True_VHAL_DrLockSta_flg : Constant  Value=TRUE  OutDataTypeStr=boolean
  True_VHAL_MIRRORFOLDSW_flg : Constant  Value=TRUE  OutDataTypeStr=boolean
  True_VHAL_RLTurnLPErr_flg : Constant  Value=TRUE  OutDataTypeStr=boolean
  True_VHAL_RLTurnLampC_mA : Constant  Value=TRUE  OutDataTypeStr=boolean
  True_VHAL_RRTurnLPErr_flg : Constant  Value=TRUE  OutDataTypeStr=boolean
  True_VHAL_RRTurnLampC_mA : Constant  Value=TRUE  OutDataTypeStr=boolean
  True_VHAL_RWiperAS_flg : Constant  Value=TRUE  OutDataTypeStr=boolean
  True_VHAL_RWiperProtection_flg : Constant  Value=TRUE  OutDataTypeStr=boolean
  slr1_{1..8} (8 alike) : BusSelector  OutputSignals=VINP_CANMsgValidZONEDR1_flg
  slr_VHAL_DrLockSta_flg : BusSelector  OutputSignals=VHAL_DrLockSta_flg
  slr_VHAL_MIRRORFOLDSW_flg : BusSelector  OutputSignals=VHAL_MIRRORFOLDSW_flg
  slr_VHAL_RLTurnLPErr_flg : BusSelector  OutputSignals=VHAL_RLTurnLPErr_flg
  slr_VHAL_RLTurnLampC_mA : BusSelector  OutputSignals=VHAL_RLTurnLampC_mA
  slr_VHAL_RRTurnLPErr_flg : BusSelector  OutputSignals=VHAL_RRTurnLPErr_flg
  slr_VHAL_RRTurnLampC_mA : BusSelector  OutputSignals=VHAL_RRTurnLampC_mA
  slr_VHAL_RWiperAS_flg : BusSelector  OutputSignals=VHAL_RWiperAS_flg
  slr_VHAL_RWiperProtection_flg : BusSelector  OutputSignals=VHAL_RWiperProtection_flg
  VINP_DrLockSta_flg : Outport
  VINP_MIRRORFOLDSW_flg : Outport  Port=2
  VINP_RLTurnLPErr_flg : Outport  Port=3
  VINP_RLTurnLampC_mA : Outport  Port=4
  VINP_RRTurnLPErr_flg : Outport  Port=5
  VINP_RRTurnLampC_mA : Outport  Port=6
  VINP_RWiperAS_flg : Outport  Port=7
  VINP_RWiperProtection_flg : Outport  Port=8
  wires:
  BHAL_outputs/1 -> [BHAL_outputs]
  inp_CanValid_bus/1 -> [inp_CanValid_bus]
  [BHAL_outputs] -> slr_VHAL_DrLockSta_flg/1
  slr_VHAL_DrLockSta_flg/1 -> DrLockSta/1  "<VHAL_DrLockSta_flg>"
  True_VHAL_DrLockSta_flg/1 -> DrLockSta/2
  [inp_CanValid_bus] -> slr1_1/1
  slr1_1/1 -> DrLockSta/3  "<VINP_CANMsgValidZONEDR1_flg>"
  DrLockSta/1 -> VINP_DrLockSta_flg/1  "VINP_DrLockSta_flg"
  DrLockSta/2 -> Terminator_1/1
  [BHAL_outputs] -> slr_VHAL_MIRRORFOLDSW_flg/1
  slr_VHAL_MIRRORFOLDSW_flg/1 -> MIRRORFOLDSW/1  "<VHAL_MIRRORFOLDSW_flg>"
  True_VHAL_MIRRORFOLDSW_flg/1 -> MIRRORFOLDSW/2
  [inp_CanValid_bus] -> slr1_2/1
  slr1_2/1 -> MIRRORFOLDSW/3  "<VINP_CANMsgValidZONEDR1_flg>"
  MIRRORFOLDSW/1 -> VINP_MIRRORFOLDSW_flg/1  "VINP_MIRRORFOLDSW_flg"
  MIRRORFOLDSW/2 -> Terminator_2/1
  [BHAL_outputs] -> slr_VHAL_RLTurnLPErr_flg/1
  slr_VHAL_RLTurnLPErr_flg/1 -> RLTurnLPErr/1  "<VHAL_RLTurnLPErr_flg>"
  True_VHAL_RLTurnLPErr_flg/1 -> RLTurnLPErr/2
  [inp_CanValid_bus] -> slr1_3/1
  slr1_3/1 -> RLTurnLPErr/3  "<VINP_CANMsgValidZONEDR1_flg>"
  RLTurnLPErr/1 -> VINP_RLTurnLPErr_flg/1  "VINP_RLTurnLPErr_flg"
  RLTurnLPErr/2 -> Terminator_3/1
  [BHAL_outputs] -> slr_VHAL_RLTurnLampC_mA/1
  slr_VHAL_RLTurnLampC_mA/1 -> RLTurnLampC/1  "<VHAL_RLTurnLampC_mA>"
  True_VHAL_RLTurnLampC_mA/1 -> RLTurnLampC/2
  [inp_CanValid_bus] -> slr1_4/1
  slr1_4/1 -> RLTurnLampC/3  "<VINP_CANMsgValidZONEDR1_flg>"
  RLTurnLampC/1 -> VINP_RLTurnLampC_mA/1  "VINP_RLTurnLampC_mA"
  RLTurnLampC/2 -> Terminator_4/1
  [BHAL_outputs] -> slr_VHAL_RRTurnLPErr_flg/1
  slr_VHAL_RRTurnLPErr_flg/1 -> RRTurnLPErr/1  "<VHAL_RRTurnLPErr_flg>"
  True_VHAL_RRTurnLPErr_flg/1 -> RRTurnLPErr/2
  [inp_CanValid_bus] -> slr1_5/1
  slr1_5/1 -> RRTurnLPErr/3  "<VINP_CANMsgValidZONEDR1_flg>"
  RRTurnLPErr/1 -> VINP_RRTurnLPErr_flg/1  "VINP_RRTurnLPErr_flg"
  RRTurnLPErr/2 -> Terminator_5/1
  [BHAL_outputs] -> slr_VHAL_RRTurnLampC_mA/1
  slr_VHAL_RRTurnLampC_mA/1 -> RRTurnLampC/1  "<VHAL_RRTurnLampC_mA>"
  True_VHAL_RRTurnLampC_mA/1 -> RRTurnLampC/2
  [inp_CanValid_bus] -> slr1_6/1
  slr1_6/1 -> RRTurnLampC/3  "<VINP_CANMsgValidZONEDR1_flg>"
  RRTurnLampC/1 -> VINP_RRTurnLampC_mA/1  "VINP_RRTurnLampC_mA"
  RRTurnLampC/2 -> Terminator_6/1
  [BHAL_outputs] -> slr_VHAL_RWiperAS_flg/1
  slr_VHAL_RWiperAS_flg/1 -> RWiperAS/1  "<VHAL_RWiperAS_flg>"
  True_VHAL_RWiperAS_flg/1 -> RWiperAS/2
  [inp_CanValid_bus] -> slr1_7/1
  slr1_7/1 -> RWiperAS/3  "<VINP_CANMsgValidZONEDR1_flg>"
  RWiperAS/1 -> VINP_RWiperAS_flg/1  "VINP_RWiperAS_flg"
  RWiperAS/2 -> Terminator_7/1
  [BHAL_outputs] -> slr_VHAL_RWiperProtection_flg/1
  slr_VHAL_RWiperProtection_flg/1 -> RWiperProtection/1  "<VHAL_RWiperProtection_flg>"
  True_VHAL_RWiperProtection_flg/1 -> RWiperProtection/2
  [inp_CanValid_bus] -> slr1_8/1
  slr1_8/1 -> RWiperProtection/3  "<VINP_CANMsgValidZONEDR1_flg>"
  RWiperProtection/1 -> VINP_RWiperProtection_flg/1  "VINP_RWiperProtection_flg"
  RWiperProtection/2 -> Terminator_8/1
